simulink model "Single_Phase_Inverter_B4"  (R2016a)
settings: Solver=VariableStepAuto  StartTime=0.0  StopTime=1  RelTol=1e-3
libraries: powerlib x8, re_lib x1
settings Model: Creator=Rangga  LastModifiedBy=Rangga

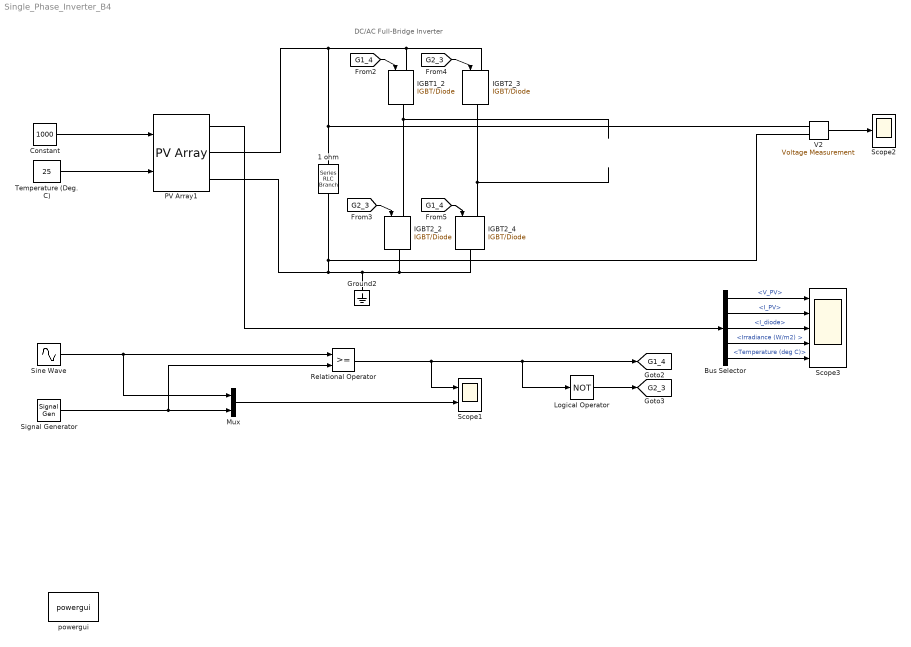
== system Single_Phase_Inverter_B4 ==
  note: DC/AC Full-Bridge Inverter
  1 ohm : powerlib/Elements/Series RLC Branch  LConnTagsString=__new0  RConnTagsString=__new0  BranchType=R  Resistance=1  Inductance=0.2e-3  SetiL0=off  InitialCurrent=0  Capacitance=[]  Setx0=off  InitialVoltage=0  Measurements=None
  Bus Selector : BusSelector  OutputSignals=V_PV,I_PV,I_diode,Irradiance (W/m2) ,Temperature (deg C)
  Constant : Constant  Value=1000
  Ground2 : powerlib/Elements/Ground  LConnTagsString=a
  IGBT1_2 : powerlib/Power Electronics/IGBT//Diode  Ron=1e-3  Rs=1e5  Cs=inf  Measurements=off
  IGBT2_2 : powerlib/Power Electronics/IGBT//Diode  Ron=1e-3  Rs=1e5  Cs=inf  Measurements=off
  IGBT2_3 : powerlib/Power Electronics/IGBT//Diode  Ron=1e-3  Rs=1e5  Cs=inf  Measurements=off
  IGBT2_4 : powerlib/Power Electronics/IGBT//Diode  Ron=1e-3  Rs=1e5  Cs=inf  Measurements=off
  Logical Operator : Logic  Operator=NOT  AllPortsSameDT=off  OutDataTypeStr=boolean
  Mux : Mux  Inputs=2
  PV Array1 : re_lib/Solar/PV Array  Npar=1  Nser=3  PlotType=one module @ 25 deg.C & specified irradiances  S_vec=1000  Temp_C_vec=[ 45 25 100 ]  ModuleName=User-defined  PlotWhenSelected=off  Pm=99.981  Ncell=36  Voc=22.5  Isc=5.75  Vm=18.9  Im=5.29  beta_Voc_pc=-0.36099  alpha_Isc_pc=0.102  beta_Voc=-0.081223  alpha_Isc=0.005865  IL=5.7584  I0=2.1256e-10  nI=1.0144  Rsh=95.9076  Rs=0.14093  BAL=on  Tc=1e-6  Tfilter=5e-5
      settings: AttributesFormatString=|
      | %<ModuleName>
      | %<Nser>-module string
      | %<Npar> parallel strings
  Relational Operator : RelationalOperator  OutDataTypeStr=boolean
  Scope1 : Scope  NumInputPorts=2
  Scope2 : Scope
  Scope3 : Scope  NumInputPorts=5
  Signal Generator : SignalGenerator  WaveForm=sawtooth  Amplitude=30  Frequency=10000  Units=rad/sec
  Sine Wave : Sin  Amplitude=20  Frequency=60*2*pi  SampleTime=0
  Temperature (Deg. C) : Constant  Value=25
  V2 : powerlib/Measurements/Voltage Measurement  Tag=PoWeRsYsTeMmEaSuReMeNt  PhasorSimulation=off  OutputType=Magnitude  PSBequivalent=0
  powergui : powerlib/powergui  Priority=1  SimulationMode=Discrete  SolverType=Tustin/Backward Euler (TBE)  SampleTime=50e-6  frequency=60  SPID=off  DisableSnubberDevices=off  DisableRonSwitches=off  DisableVfSwitches=off  SwTol=0  DisplayEquations=off  Interpol=off  ExternalGateDelay=off  methode=off  Ts=10  FunctionMessages=off  echomessages=off  HookPort=off  EnableUseOfTLC=off  x0status=blocks  frequencyindice=0  Pbase=100e6  ErrMax=1e-4  Iterations=50  UnitsV=kV  UnitsW=MW  buscounter=0  RestoreLinks=warning  ResistiveCurrentMeasurement=off  Frange=[0:2:500]  Ylog=off  Xlog=on  ShowGrid=off  save=off  variable=ZData  structure=0  ZoomFFT=off  StartTime=0.0  cycles=1  DisplayStyle=1  fundamental=60  FreqAxis=off  MaxFrequency=1000  frequencyindicesteady=1  RmsSteady=1  display=off
  tag scope: G1_4=global, G2_3=global
  wires:
  [G1_4] -> IGBT1_2/1
  [G2_3] -> IGBT2_2/1
  [G2_3] -> IGBT2_3/1
  [G1_4] -> IGBT2_4/1
  Signal Generator/1 -> Mux/2, Relational Operator/2
  Relational Operator/1 -> Scope1/1, Logical Operator/1, [G1_4]
  Logical Operator/1 -> [G2_3]
  Sine Wave/1 -> Mux/1, Relational Operator/1
  Mux/1 -> Scope1/2
  V2/1 -> Scope2/1
  Constant/1 -> PV Array1/1
  Temperature (Deg. C)/1 -> PV Array1/2
  Bus Selector/1 -> Scope3/1  "<V_PV>"
  Bus Selector/2 -> Scope3/2  "<I_PV>"
  Bus Selector/3 -> Scope3/3  "<I_diode>"
  Bus Selector/4 -> Scope3/4  "<Irradiance (W/m2) >"
  Bus Selector/5 -> Scope3/5  "<Temperature (deg C)>"
  PV Array1/1 -> Bus Selector/1
  connections:
  IGBT2_2/RConn1 -- IGBT2_4/RConn1 -- 1 ohm/RConn1 -- V2/LConn2 -- PV Array1/RConn2 -- Ground2/LConn1
  IGBT1_2/LConn1 -- 1 ohm/LConn1 -- V2/LConn1 -- PV Array1/RConn1 -- IGBT2_3/LConn1
  IGBT1_2/RConn1 -- IGBT2_2/LConn1
  IGBT2_3/RConn1 -- IGBT2_4/LConn1
